simulink model "Kin_v_Sek_cc"  (R2015b)
settings: Solver=FixedStepDiscrete  StartTime=0.0  StopTime=10  FixedStep=0.010  RelTol=1e-3
PostLoadFcn:
  | , if any(exist('dsrtsu_mdlpostloadfcn', 'file') == [2, 3, 6]), try dsrtsu_mdlpostloadfcn('Execute', bdroot); catch fprintf('Error in PostLoadFcn (dsrtsu_mdlpostloadfcn) for model "%s":\n %s\n', bdroot, lasterr); end, end,
values from neighbouring files (symbols this model uses):
  ii = 1    [PAR_Kin_v_Sek_cc.m]
undefined symbols (not defined in the file or in its folder): BHA, DiscIntNeverNeededParam, lData
libraries: libo_robotics x1
settings Model: DSRTSU_INTERNAL_RTI_VER=440  DSRTSU_INTERNAL_RTI_TYPE=rti1007  DSRTSU_INTERNAL_RTIFPGA=30  Creator=Mahl  LastModifiedBy=Mayer
settings DataIOCC: SaveFormat=Array  SignalLoggingSaveFormat=ModelDataLogs
settings OptimizationCC: BlockReduction=off  OptimizeBlockIOStorage=off  BufferReuse=off  GlobalBufferReuse=off  ExpressionFolding=off  ExpressionDepthLimit=2147483647  LocalBlockOutputs=off
settings DebuggingCC: UnderspecifiedInitializationDetection=Classic  MergeDetectMultiDrivingBlocksExec=none  SolverPrmCheckMsg=warning  FcnCallInpInsideContextMsg=UseLocalSettings  StateNameClashWarn=warning
settings HardwareCC: ProdBitPerPointer=32  ProdLargestAtomicFloat=None  ProdEndianess=BigEndian  ProdWordSize=32  ProdHWDeviceType=Generic->Custom  TargetIntDivRoundTo=Zero  TargetEndianess=BigEndian  TargetHWDeviceType=Generic->Custom
settings RTWCC: SystemTargetFile=rti1103.tlc  MakeCommand=make_rti  TemplateMakefile=rti1103.tmf  Description=dSPACE DS1103 Hardware Platform
settings STFCustomTargetCC: ParMdlRefBuildCompliant=on  ConcurrentExecutionCompliant=off  MatFileLogging=on  SystemTargetFile=rti1103.tlc
settings GRTTargetCC: CompOptLevelCompliant=off  ConcurrentExecutionCompliant=off  GeneratePreprocessorConditionals=Disable all  CombineOutputUpdateFcns=off  GRTInterface=on  UseToolchainInfoCompliant=off  ExtModeMexFile=noextcomm
settings ConfigComp: CovModelRefEnable=Off

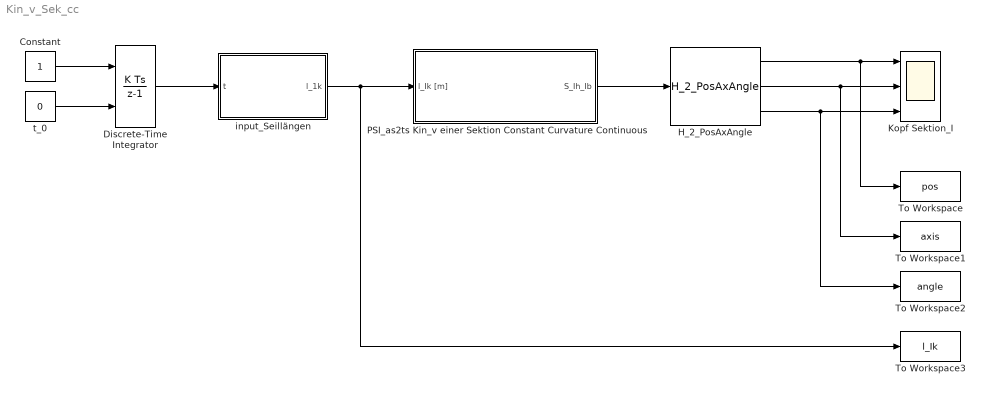
== system Kin_v_Sek_cc ==
  Constant : Constant
  Discrete-Time Integrator : DiscreteIntegrator  InitialConditionSource=external  SampleTime=0.010  ICPrevOutput=DiscIntNeverNeededParam  ICPrevScaledInput=DiscIntNeverNeededParam
  H_2_PosAxAngle : libo_robotics/Kinematics/H_2_PosAxAngle
  Kopf Sektion_I : Scope  NumInputPorts=3
  PSI_as2ts Kin_v einer Sektion Constant Curvature Continuous : Subsystem  mask{ii=ii}
      mask prompts: ii "Sektionsnummer"
      mask help:
      | -- Vorwärtskinematik einer Sektion des BHAs --
      |
      | Wahl der Sektionsnummer:
      | 1 = groß
      | 2 = mittel
      | 3 = klein
      settings: AttributesFormatString=ii = %<ii>
  To Workspace : ToWorkspace  VariableName=pos  SaveFormat=Structure With Time  SampleTime=-1
      settings: Decimation=10
  To Workspace1 : ToWorkspace  VariableName=axis  SaveFormat=Structure With Time  SampleTime=-1
      settings: Decimation=10
  To Workspace2 : ToWorkspace  VariableName=angle  SaveFormat=Structure With Time  SampleTime=-1
      settings: Decimation=10
  To Workspace3 : ToWorkspace  VariableName=l_Ik  SaveFormat=Structure With Time  SampleTime=-1
      settings: Decimation=10
  input_Seillängen : Subsystem
  t_0 : Constant  Value=0
  wires:
  input_Seillängen/1(l_1k) -> PSI_as2ts Kin_v einer Sektion Constant Curvature Continuous/1(l_Ik [m]), To Workspace3/1
  Discrete-Time Integrator/1 -> input_Seillängen/1(t)
  Constant/1 -> Discrete-Time Integrator/1
  t_0/1 -> Discrete-Time Integrator/2
  PSI_as2ts Kin_v einer Sektion Constant Curvature Continuous/1(S_Ih_Ib) -> H_2_PosAxAngle/1
  H_2_PosAxAngle/1 -> Kopf Sektion_I/1, To Workspace/1
  H_2_PosAxAngle/2 -> Kopf Sektion_I/2, To Workspace1/1
  H_2_PosAxAngle/3 -> Kopf Sektion_I/3, To Workspace2/1

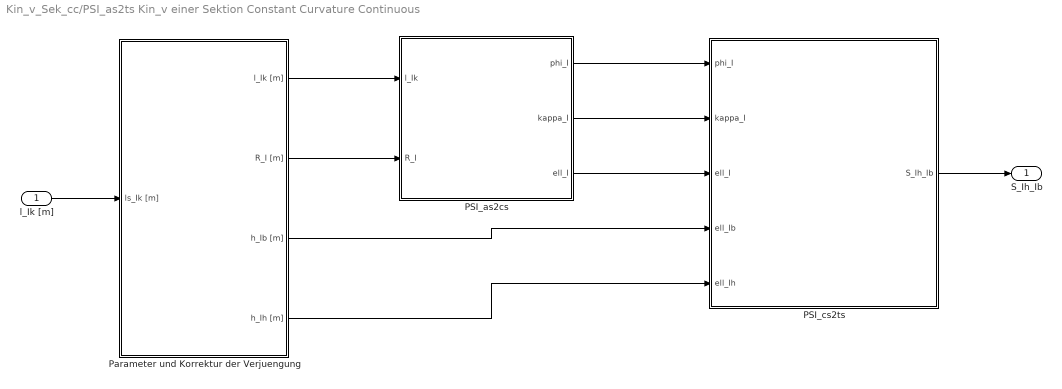
== system Kin_v_Sek_cc/PSI_as2ts Kin_v einer Sektion Constant Curvature Continuous ==
  l_Ik [m] : Inport
  PSI_as2cs : Subsystem
  PSI_cs2ts : MATLAB Function  TreatAsAtomicUnit=on
  Parameter und Korrektur der Verjuengung : Subsystem
  S_Ih_Ib : Outport
  wires:
  l_Ik [m]/1 -> Parameter und Korrektur der Verjuengung/1(ls_Ik [m])
  Parameter und Korrektur der Verjuengung/1(l_Ik [m]) -> PSI_as2cs/1(l_Ik)
  Parameter und Korrektur der Verjuengung/2(R_I [m]) -> PSI_as2cs/2(R_I)
  PSI_as2cs/1(phi_I) -> PSI_cs2ts/1(phi_I)
  PSI_as2cs/2(kappa_I) -> PSI_cs2ts/2(kappa_I)
  PSI_as2cs/3(ell_I) -> PSI_cs2ts/3(ell_I)
  PSI_cs2ts/1(S_Ih_Ib) -> S_Ih_Ib/1
  Parameter und Korrektur der Verjuengung/3(h_Ib [m]) -> PSI_cs2ts/4(ell_Ib)
  Parameter und Korrektur der Verjuengung/4(h_Ih [m]) -> PSI_cs2ts/5(ell_Ih)

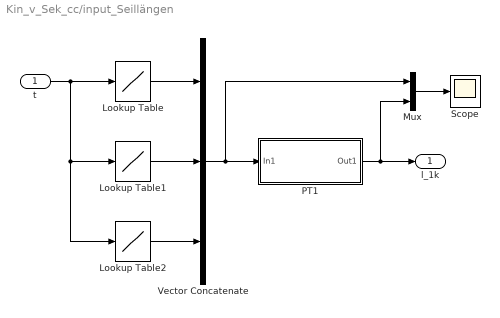
== system Kin_v_Sek_cc/input_Seillängen ==
  t : Inport
  Lookup Table : Lookup  InputValues=lData.time  Table=lData.l_1k(1,:)  LookUpMeth=Use Input Nearest
      settings: AttributesFormatString=%<Table>
  Lookup Table1 : Lookup  InputValues=lData.time  Table=lData.l_1k(2,:)  LookUpMeth=Use Input Nearest
      settings: AttributesFormatString=%<Table>
  Lookup Table2 : Lookup  InputValues=lData.time  Table=lData.l_1k(3,:)  LookUpMeth=Use Input Nearest
      settings: AttributesFormatString=%<Table>
  Mux : Mux  Inputs=2
  PT1 : Subsystem
  Scope : Scope
  Vector Concatenate : Concatenate  NumInputs=3  Mode=Multidimensional array
  l_1k : Outport
  wires:
  t/1 -> Lookup Table2/1, Lookup Table1/1, Lookup Table/1
  Lookup Table/1 -> Vector Concatenate/1
  Lookup Table1/1 -> Vector Concatenate/2
  Lookup Table2/1 -> Vector Concatenate/3
  Vector Concatenate/1 -> PT1/1(In1), Mux/1
  PT1/1(Out1) -> l_1k/1, Mux/2
  Mux/1 -> Scope/1

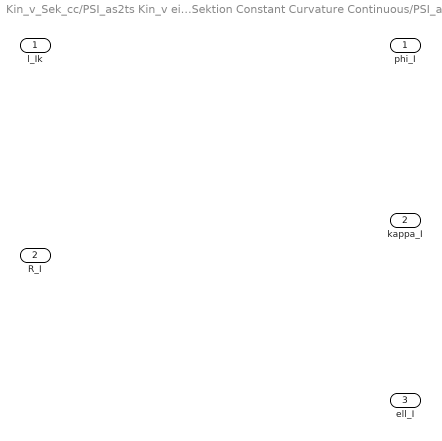
== system Kin_v_Sek_cc/PSI_as2ts Kin_v einer Sektion Constant Curvature Continuous/PSI_as2cs ==
  l_Ik : Inport
  R_I : Inport  Port=2
  phi_I : Outport
  kappa_I : Outport  Port=2
  ell_I : Outport  Port=3

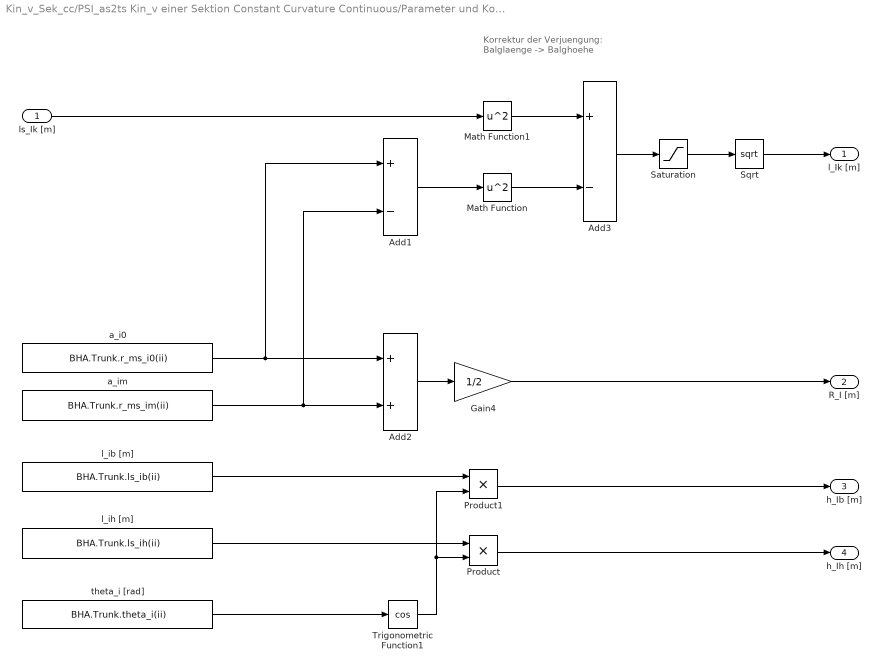
== system Kin_v_Sek_cc/PSI_as2ts Kin_v einer Sektion Constant Curvature Continuous/Parameter und Korrektur der Verjuengung ==
  note: Korrektur der Verjuengung:
      | Balglaenge -> Balghoehe
  ls_Ik [m] : Inport
  Add1 : Sum  Inputs=+-
  Add2 : Sum
  Add3 : Sum  Inputs=+-
  Gain4 : Gain  Gain=1/2
  Math Function : Math  Operator=square  SaturateOnIntegerOverflow=on
  Math Function1 : Math  Operator=square  SaturateOnIntegerOverflow=on
  Product : Product  RndMeth=Zero
  Product1 : Product  RndMeth=Zero
  Saturation : Saturate  UpperLimit=inf  LowerLimit=0
  Sqrt : Sqrt  SaturateOnIntegerOverflow=on
  Trigonometric Function1 : Trigonometry  Operator=cos
  a_i0 : Constant  Value=BHA.Trunk.r_ms_i0(ii)  VectorParams1D=off
  a_im : Constant  Value=BHA.Trunk.r_ms_im(ii)  VectorParams1D=off
  l_ib [m] : Constant  Value=BHA.Trunk.ls_ib(ii)  VectorParams1D=off
  l_ih [m] : Constant  Value=BHA.Trunk.ls_ih(ii)  VectorParams1D=off
  theta_i [rad] : Constant  Value=BHA.Trunk.theta_i(ii)  VectorParams1D=off
  l_Ik [m] : Outport
  R_I [m] : Outport  Port=2
  h_Ib [m] : Outport  Port=3
  h_Ih [m] : Outport  Port=4
  wires:
  Sqrt/1 -> l_Ik [m]/1
  Saturation/1 -> Sqrt/1
  Math Function/1 -> Add3/2
  Math Function1/1 -> Add3/1
  Add1/1 -> Math Function/1
  Trigonometric Function1/1 -> Product1/2, Product/2
  ls_Ik [m]/1 -> Math Function1/1
  Add3/1 -> Saturation/1
  Product1/1 -> h_Ib [m]/1
  Product/1 -> h_Ih [m]/1
  Add2/1 -> Gain4/1
  Gain4/1 -> R_I [m]/1
  l_ib [m]/1 -> Product1/1
  l_ih [m]/1 -> Product/1
  theta_i [rad]/1 -> Trigonometric Function1/1
  a_i0/1 -> Add1/1, Add2/1
  a_im/1 -> Add1/2, Add2/2

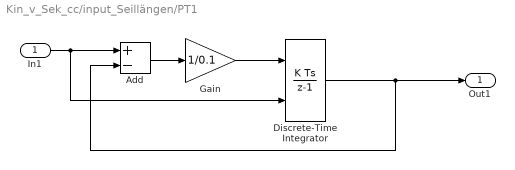
== system Kin_v_Sek_cc/input_Seillängen/PT1 ==
  In1 : Inport
  Add : Sum  Inputs=+-
  Discrete-Time Integrator : DiscreteIntegrator  InitialConditionSource=external  SampleTime=0.010  ICPrevOutput=DiscIntNeverNeededParam  ICPrevScaledInput=DiscIntNeverNeededParam
  Gain : Gain  Gain=1/0.1
  Out1 : Outport
  wires:
  In1/1 -> Add/1, Discrete-Time Integrator/2
  Add/1 -> Gain/1
  Discrete-Time Integrator/1 -> Out1/1, Add/2
  Gain/1 -> Discrete-Time Integrator/1

== matlab function Kin_v_Sek_cc/PSI_as2ts Kin_v einer Sektion Constant Curvature Continuous/PSI_cs2ts ==
  data: phi_I input; S_Ih_Ib output; kappa_I input; ell_I input; ell_Ib input; ell_Ih input
function S_Ih_Ib = PSI_cs2ts(phi_I, kappa_I, ell_I, ell_Ib, ell_Ih)

% Berechnung der homogenen Transformation der I-ten Sektion gemäß Abbildung
% PSI_cs2ts(phi_I, kappa_I, ell_I)
% 
% Input:    Konfigurationszustand
% Output:   homogene Transformation zwischen Kopf- und Fuß-Koordinatensystem

%% homogene Transformation des Fußes
U_I0_Ib = [eye(3), [0; 0; ell_Ib];...
           0,0,0,  1];

%% homogene Transformation des Kopfs
U_Ih_I1 = [eye(3), [0; 0; ell_Ih];...
           0,0,0,  1];

%% homogene Transformation des Aktorbereichs
eps =   1e-7;

% Berechnung gemäß lim kappa->0 (Biegelinie ist eine Gerade)
if(kappa_I < eps)
    C_I1_I0 = eye(3);
    O_I1_I0 = [0; 0; ell_I];

% Berechnung gemäß kappa>0 (Biegelinie ist ein Kreissegment)
else
    s_phi   = sin(phi_I);
    c_phi   = cos(phi_I);
    s_kl    = sin(kappa_I*ell_I);
    c_kl    = cos(kappa_I*ell_I);
    
    C_I1_I0 = [c_phi^2*(c_kl-1)+1,      s_phi*c_phi*(c_kl-1),       c_phi*s_kl;...
               s_phi*c_phi*(c_kl-1),    c_phi^2*(1-c_kl)+c_kl,      s_phi*s_kl;...
               -c_phi*s_kl,             -s_phi*s_kl,                c_kl];
           
    O_I1_I0 = [c_phi*(1-c_kl)/kappa_I;...
               s_phi*(1-c_kl)/kappa_I;...
               s_kl/kappa_I];
end
U_I1_I0 = [C_I1_I0, O_I1_I0;...
           0,0,0,   1];
       
S_Ih_Ib = U_I0_Ib*U_I1_I0*U_Ih_I1;
